simulink model "NeuronalNetwork"  (R2019b)
settings: Solver=VariableStepAuto  StartTime=0.0  StopTime=10.0  RelTol=1e-3
libraries: neural x1006
(part 2 of 11)

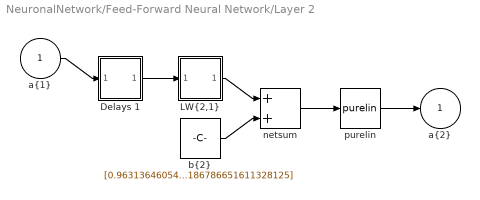
== system NeuronalNetwork/Feed-Forward Neural Network/Layer 2 ==
  "a{1} " : Inport  PortDimensions=1  SampleTime=0.1
      mask Display: e = 0.06;c1 = [120 230 180]/255;c2 = ([120 230 180]+0)/(256+128);c3 = ([120 230 180]+128)/(256+128);patch([0 1 1 0],[0 0 1 1],c1);patch([0 1 1 1-e 1-e 0+e],[0 0 1 1-e 0+e 0+e],c2);patch([0 0 1 1-e 0+e 0+e],[0 1 1 1-e 1-e 0+e],c3);plot([0 1 1 0 0],[0 0 1 1 0]);
  Delays 1 : Subsystem
      mask Display: e = 0.06;c1 = [120 150 230]/255;c2 = ([120 150 230]+0)/383;c3 = ([120 150 230]+128)/383;patch([0 1 1 0],[0 0 1 1],c1);patch([0 1 1 1-e 1-e 0+e],[0 0 1 1-e 0+e 0+e],c2);patch([0 0 1 1-e 0+e 0+e],[0 1 1 1-e 1-e 0+e],c3);plot([0 1 1 0 0],[0 0 1 1 0]);disp('0');
  "LW{2,1}" : Subsystem
      mask Display: e = 0.06;c1 = [120 150 230]/255;c2 = ([120 150 230]+0)/383;c3 = ([120 150 230]+128)/383;patch([0 1 1 0],[0 0 1 1],c1);patch([0 1 1 1-e 1-e 0+e],[0 0 1 1-e 0+e 0+e],c2);patch([0 0 1 1-e 0+e 0+e],[0 1 1 1-e 1-e 0+e],c3);plot([0 1 1 0 0],[0 0 1 1 0]);disp('W');
  "b{2}" : Constant  Value=[0.9631364605458718752828417564160190522670745849609375;-0.8195154219681992646684420833480544388294219970703125;0.3723173165774313897458114297478459775447845458984375;0.85792960258715478261137832305394113063812255859375;-0.71636725809811796494841473759151995182037353515625;0.7688313075261010709482434322126209735870361328125;-0.960476077419632812137706423527561128139495849609375;-0.3146282067465147047613527320208959281444549560546875;-0.5233878248982624104002070453134365379810333251953125;0.9691280019260635203437459495035000145435333251953125;0.693195804234663537357619134127162396907806396484375;0.589023192789889460385666097863577306270599365234375;0.800556133365972311111136150429956614971160888671875;0.5602094374445873992129918406135402619838714599609375;0.673021543293496282700516530894674360752105712890625;-0.357813471110595582302948969299905002117156982421875;0.4854911518033400152916101433220319449901580810546875;0.328988569993101886979047776549123227596282958984375;-0.4216326187959331672772123056347481906414031982421875;-0.3252555340443930020910556777380406856536865234375;0.8172741183508802631507705882540903985500335693359375;-0.9354980391174045895041899711941368877887725830078125;0.392715455911331279281739625730551779270172119140625;-0.5824603682222215805808218647143803536891937255859375;0.6482987126558714674473549166577868163585662841796875;-0.563535472532050274452330995700322091579437255859375;-0.8007153940767726130189885225263424217700958251953125;0.2390116328916460641806907005957327783107757568359375;-0.7923704346977882284619454367202706634998321533203125;0.5981236071792732644780699047259986400604248046875;0.805850238565878118635055216145701706409454345703125;-0.3749743080266665362643152548116631805896759033203125;-0.4368216676815526167132475165999494493007659912109375;-0.9864361174638818230420156396576203405857086181640625;-0.0082566686664284905106114820227958261966705322265625;0.9769644860245738637871681930846534669399261474609375;0.4758815029910381522171292090206407010555267333984375;-0.37856036521686053930579873849637806415557861328125;0.2008150007023010719109379351721145212650299072265625;0.5633596533222309243882364171440713107585906982421875;-0.7769337506301134954611598004703409969806671142578125;0.158658578777811865023750215186737477779388427734375;0.7407424406234397462611696028034202754497528076171875;0.3795524992222478743997271521948277950286865234375;-0.514059498156742566976618036278523504734039306640625;-0.314555496260482403414471264113672077655792236328125;0.0908795759508513878444091460551135241985321044921875;-0.86485461462136736798811398330144584178924560546875;-0.1791032006029109613365335462731309235095977783203125;-0.5249772055412129656559727663989178836345672607421875;-0.0220528871505454304724480607546865940093994140625;0.612133176603574913343663865816779434680938720703125;-0.24430409665764241111673982231877744197845458984375;0.035956289014776654511251763324253261089324951171875;-0.8108042213100967732231083573424257338047027587890625;0.818190385699671285379963592276908457279205322265625;-0.5847388120053158555577965671545825898647308349609375;-0.235870952918940446352280559949576854705810546875;0.3205605303573701991837197056156583130359649658203125;0.5167466045551443176719885741476900875568389892578125;-0.6538611752158078882501968109863810241222381591796875;0.0347595230126518384139444606262259185314178466796875;0.990676224606932276373072454589419066905975341796875;0.41521881318141762307050157687626779079437255859375;-0.8388653981521383418140658250194974243640899658203125;-0.913383807249795065530406645848415791988372802734375;-0.0176888740314791181873488312703557312488555908203125;-0.106807119661594729365106104523874819278717041015625;-0.02640286830930893557933814008720219135284423828125;-0.668217755829316306659393376321531832218170166015625;-0.2786869903737765330475895098061300814151763916015625;0.7614438835274268679853548746905289590358734130859375;0.4887043599923990289113362450734712183475494384765625 ...(+50519 chars)]
      mask Display: e = 0.06;c1 = [120 150 230]/255;c2 = ([120 150 230]+0)/383;c3 = ([120 150 230]+128)/383;patch([0 1 1 0],[0 0 1 1],c1);patch([0 1 1 1-e 1-e 0+e],[0 0 1 1-e 0+e 0+e],c2);patch([0 0 1 1-e 0+e 0+e],[0 1 1 1-e 1-e 0+e],c3);plot([0 1 1 0 0],[0 0 1 1 0]);disp('b');
  netsum : Sum  Inputs=2  SaturateOnIntegerOverflow=on  InputSameDT=on  OutDataTypeStr=Inherit: Same as first input
      mask Display: e = 0.06;c1 = [120 150 230]/255;c2 = ([120 150 230]+0)/383;c3 = ([120 150 230]+128)/383;patch([0 1 1 0],[0 0 1 1],c1);patch([0 1 1 1-e 1-e 0+e],[0 0 1 1-e 0+e 0+e],c2);patch([0 0 1 1-e 0+e 0+e],[0 1 1 1-e 1-e 0+e],c3);plot([0 1 1 0 0],[0 0 1 1 0]);disp('+');
  purelin : neural/Transfer Functions/purelin
      settings: SourceProductName=Deep Learning Toolbox
  "a{2}" : Outport  InitialOutput=[0;0;0;0;0;0;0;0;0;0;0;0;0;0;0;0;0;0;0;0;0;0;0;0;0;0;0;0;0;0;0;0;0;0;0;0;0;0;0;0;0;0;0;0;0;0;0;0;0;0;0;0;0;0;0;0;0;0;0;0;0;0;0;0;0;0;0;0;0;0;0;0;0;0;0;0;0;0;0;0;0;0;0;0;0;0;0;0;0;0;0;0;0;0;0;0;0;0;0;0;0;0;0;0;0;0;0;0;0;0;0;0;0;0;0;0;0;0;0;0;0;0;0;0;0;0;0;0;0;0;0;0;0;0;0;0;0;0;0;0;0;0;0;0;0;0;0;0;0;0;0;0;0;0;0;0;0;0;0;0;0;0;0;0;0;0;0;0;0;0;0;0;0;0;0;0;0;0;0;0;0;0;0;0;0;0;0;0;0;0;0;0;0;0;0;0;0;0;0;0;0;0;0;0;0;0;0;0;0;0;0;0;0;0;0;0;0;0;0;0;0;0;0;0;0;0;0;0;0;0;0;0;0;0;0;0;0;0;0;0;0;0;0;0;0;0;0;0;0;0;0;0;0;0;0;0;0;0;0;0;0;0;0;0;0;0;0;0;0;0;0;0;0;0;0;0;0;0;0;0;0;0;0;0;0;0;0;0;0;0;0;0;0;0;0;0;0;0;0;0;0;0;0;0;0;0;0;0;0;0;0;0;0;0;0;0;0;0;0;0;0;0;0;0;0;0;0;0;0;0;0;0;0;0;0;0;0;0;0;0;0;0;0;0;0;0;0;0;0;0;0;0;0;0;0;0;0;0;0;0;0;0;0;0;0;0;0;0;0;0;0;0;0;0;0;0;0;0;0;0;0;0;0;0;0;0;0;0;0;0;0;0;0;0;0;0;0;0;0;0;0;0;0;0;0;0;0;0;0;0;0;0;0;0;0;0;0;0;0;0;0;0;0;0;0;0;0;0;0;0;0;0;0;0;0;0;0;0;0;0;0;0;0;0;0;0;0;0;0;0;0;0;0;0;0;0;0;0;0;0;0;0;0;0;0;0;0;0;0;0;0;0;0;0;0;0;0;0;0;0;0;0;0;0;0;0;0;0;0;0;0;0;0;0;0;0;0;0;0;0;0;0;0;0;0;0;0;0;0;0;0;0;0;0;0;0;0;0;0;0;0;0;0;0;0;0;0;0;0;0;0;0;0;0;0;0;0;0;0;0;0;0;0;0;0;0;0;0;0;0;0;0;0;0;0;0;0;0;0;0;0;0;0;0;0;0;0;0;0;0;0;0;0;0;0;0;0;0;0;0;0;0;0;0;0;0;0;0;0;0;0;0;0;0;0;0;0;0;0;0;0;0;0;0;0;0;0;0;0;0;0;0;0;0;0;0;0;0;0;0;0;0;0;0;0;0;0;0;0;0;0;0;0;0;0;0;0;0;0;0;0;0;0;0;0;0;0;0;0;0;0;0;0;0;0;0;0;0;0;0;0;0;0;0;0;0;0;0;0;0;0;0;0;0;0;0;0;0;0;0;0;0;0;0;0;0;0;0;0;0;0;0;0;0;0;0;0;0;0;0;0;0;0;0;0;0;0;0;0;0;0;0;0;0;0;0;0;0;0;0;0;0;0;0;0;0;0;0;0;0;0;0;0;0;0;0;0;0;0;0;0;0;0;0;0;0;0;0;0;0;0;0;0;0;0;0;0;0;0;0;0;0;0;0;0;0;0;0;0;0;0;0;0;0;0;0;0;0;0;0;0;0;0;0;0;0;0;0;0;0;0;0;0;0;0;0;0;0;0;0;0;0;0;0;0;0;0;0;0;0;0;0;0;0;0;0;0;0;0;0;0;0;0;0;0;0;0;0;0;0;0;0;0;0;0;0;0;0;0;0;0;0;0;0;0;0;0;0;0;0;0;0;0;0;0;0;0;0;0;0;0;0;0;0;0;0;0;0;0;0;0;0;0;0;0;0;0;0;0;0;0;0;0;0;0;0;0;0;0;0;0;0;0;0;0;0;0;0;0;0;0;0;0;0;0;0;0;0;0;0;0;0;0;0;0;0;0;0;0;0;0;0;0;0;0;0;0;0;0;0;0;0;0;0;0;0;0;0;0;0;0;0;0;0;0;0;0;0;0;0;0;0;0;0;0;0;0;0;0;0;0;0;0;0;0;0;0;0;0;0;0;0;0;0;0;0;0;0;0;0;0;0;0;0;0;0;0;0;0;0;0;0;0;0;0;0;0;0;0;0;0]
      mask Display: e = 0.06;c1 = [120 230 180]/255;c2 = ([120 230 180]+0)/(256+128);c3 = ([120 230 180]+128)/(256+128);patch([0 1 1 0],[0 0 1 1],c1);patch([0 1 1 1-e 1-e 0+e],[0 0 1 1-e 0+e 0+e],c2);patch([0 0 1 1-e 0+e 0+e],[0 1 1 1-e 1-e 0+e],c3);plot([0 1 1 0 0],[0 0 1 1 0]);
  wires:
  "a{1} "/1 -> Delays 1/1("p{2}")
  Delays 1/1("pd{2,1}") -> "LW{2,1}"/1("ad{2,1}")
  "LW{2,1}"/1("lz{2,1}") -> netsum/1
  "b{2}"/1 -> netsum/2
  netsum/1 -> purelin/1
  purelin/1 -> "a{2}"/1
